simulink model "AMR_main_model_23b"  (R2023b)
settings: Solver=FixedStepAuto  StartTime=0.0  StopTime=inf  RelTol=1e-3
model workspace (MAT data in the model file):
  RTK_health_condition = 30
  mdlWSDbList = ["C:\Users\matlab.cut\Desktop\AMR\canbus_files\tramontina_database_mobotic.dbc" "C:\Users\matlab.cut\Desktop\AMR\canbus_files\tramontina_database_nvidia.dbc" "C:\Users\matlab.cut\Desktop\AMR\canbus_files\tramontina_database_sick_modbus.dbc" "C:\Users\matlab.cut\Desktop\AMR\canbus_files\tramontina_database_xsens.dbc" "tramontina_database_curtis.dbc"]
  min_motor_rpm = 30
  wheel_diameter = 360
undefined symbols (not defined in the file or in its folder): Down, Pull
libraries: speedgoatlib_IO60X_IO69X x12, tramontina_database_nvidialib x7, tramontina_database_curtislib x7, tramontina_database_xsenslib x4, speedgoatlib_IO691 x2, simulink x2, tramontina_database_sick_modbuslib x1, canmsglib x1
(part 1 of 2)
settings Model: Creator=matlab.cut  LastModifiedBy=matlab.cut
settings SolverCC: ConcurrentTasks=on  PositivePriorityOrder=on
settings OptimizationCC: BlockReduction=off  OptimizeBlockIOStorage=off
settings DebuggingCC: TasksWithSamePriorityMsg=none
settings HardwareCC: ProdBitPerLong=64  ProdLongLongMode=on  ProdHWDeviceType=Intel->x86-64 (Linux 64)
settings SFSimCC: MATLABDynamicMemAlloc=off
settings RTWCC: Description=Simulink Real-Time  SystemTargetFile=slrealtime.tlc  TemplateMakefile=slrealtime_default_tmf  Toolchain=Simulink Real-Time Toolchain  BuildConfiguration=Faster Runs  CodeExecutionProfiling=on  TargetLang=C++
settings CodeAppCC: MaxIdLength=127

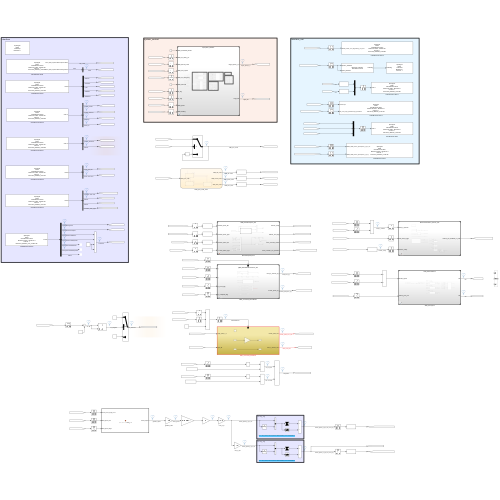
[thumbnail: Simulink's stored preview of the top-level diagram]
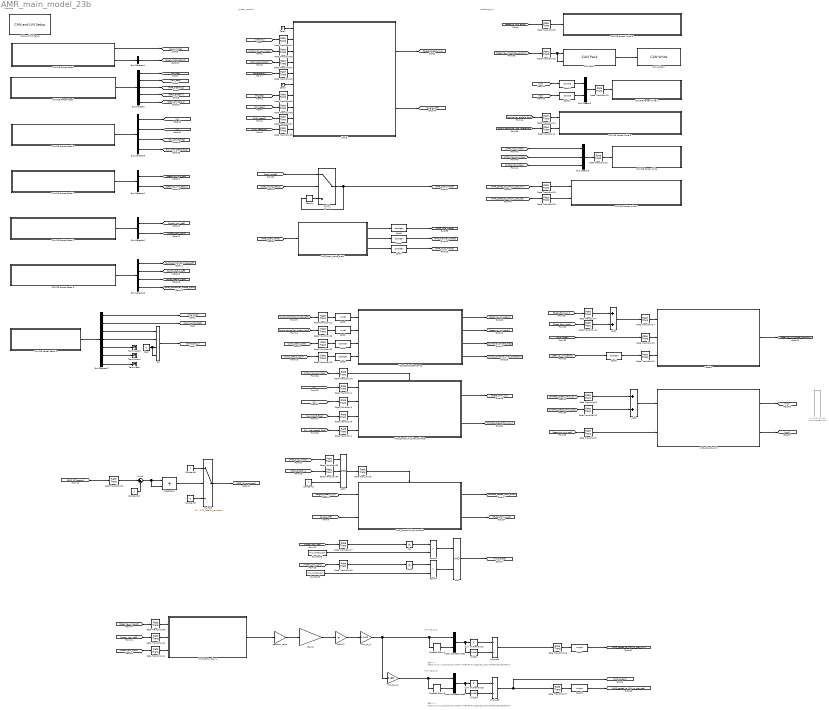
== system AMR_main_model_23b ==
  note: interface
  note: system_control
  note: interface_out
  note: REF ->> https://www.youtube.com/watch?v=BV3H-0wlcSs&ab_channel=EmbeddedRoom
  note: moving_avg
  note: REF ->> https://www.youtube.com/watch?v=BV3H-0wlcSs&ab_channel=EmbeddedRoom
  note: moving_avg
  AMR_ControlUnit_AutoMode : Subsystem  TreatAsAtomicUnit=on
  AMR_ControlUnit_ManualMode : ModelReference  ModelNameDialog=AMR_ManualModeControlUnit_23b.slx  SimulationMode=Normal  ModelReferenceVersion=1.33  EnablePortName=Enable  EnablePortStatesWhenEnabling=held
  AMR_VelocityUnit : ModelReference  ModelNameDialog=AMR_differentialDrive.slx  SimulationMode=Normal  ModelReferenceVersion=1.13
  AMR_oper_mode_chart : Stateflow chart  TreatAsAtomicUnit=on
  AND : Logic  AllPortsSameDT=off  OutDataTypeStr=boolean
  AND1 : Logic  Inputs=3  AllPortsSameDT=off  OutDataTypeStr=boolean
  Abs : Abs  SaturateOnIntegerOverflow=off
  Abs3 : Abs  SaturateOnIntegerOverflow=off
  Add1 : Sum
  Add2 : Sum
  Bus Creator2 : BusCreator  Inputs=2
  Bus Creator3 : BusCreator  Inputs=3
  Bus Selector : BusSelector  OutputSignals=ID113_LongLat.latitude,ID113_LongLat.longitude,ID34_EulerAngles.yaw,ID17_StatusWord.GNSSfix,ID17_StatusWord.RtkStatus
  Bus Selector1 : BusSelector  OutputSignals=ID288_mobotic_feedback_pos.position_feedback,ID288_mobotic_feedback_pos.MessageStatus.Status
  Bus Selector2 : BusSelector  OutputSignals=ID422_curtis_feedback_message_left.motor_rpm_left,ID423_curtis_feedback_message_right.motor_rpm_right
  Bus Selector4 : BusSelector  OutputSignals=Status  OutputAsBus=on
  Bus Selector5 : BusSelector  OutputSignals=ID368_joystick_axes.joystick_throttle,ID368_joystick_axes.joystick_direction,ID369_joystick_buttons.button_5,ID369_joystick_buttons.button_6
  Bus Selector6 : BusSelector  OutputSignals=ID1830_controller_status_left.controller_mode_left,ID1830_controller_status_left.MessageStatus.Status,ID1831_controller_status_right.MessageStatus.Status,ID1831_controller_status_right.controller_mode_right
  Bus Selector7 : BusSelector  OutputSignals=ID341_read_from_flexisoft.AuxEmEmergencia,ID341_read_from_flexisoft.AuxScannerInterrompido,ID341_read_from_flexisoft.EmergenciaFrontalDireita,ID341_read_from_flexisoft.EmergenciaFrontalEsquerda,ID341_read_from_flexisoft.EmergenciaTraseiraDireita,ID341_read_from_flexisoft.EmergenciaTraseiraEsquerda,ID341_read_from_flexisoft.MessageStatus.Status
  CAN DB Parser Read : Subsystem
      settings: OpenFcn=sg_can.OpenFcnRead;
      mask Help: eval('sg.utils.help.show(''io_main/refentry_ref_can_ofa_parsing_read'');')
      mask Display: disp('Speedgoat\nIO691\nCAN DB Parser Read\nModule ID: IO691 - Module ID 1\nChannel:  1\ntramontina_database_xsens.dbc ');
  "CAN DB Parser Read " : Subsystem
      settings: OpenFcn=sg_can.OpenFcnRead;
      mask Help: eval('sg.utils.help.show(''io_main/refentry_ref_can_ofa_parsing_read'');')
      mask Display: disp('Speedgoat\nIO691\nCAN DB Parser Read\nModule ID: IO691 - Module ID 1\nChannel:  1\ntramontina_database_nvidia.dbc ');
  CAN DB Parser Read 1 : Subsystem
      settings: OpenFcn=sg_can.OpenFcnRead;
      mask Help: eval('sg.utils.help.show(''io_main/refentry_ref_can_ofa_parsing_read'');')
      mask Display: disp('Speedgoat\nIO691\nCAN DB Parser Read\nModule ID: IO691 - Module ID 1\nChannel:  1\ntramontina_database_nvidia.dbc ');
  CAN DB Parser Read 2 : Subsystem
      settings: OpenFcn=sg_can.OpenFcnRead;
      mask Help: eval('sg.utils.help.show(''io_main/refentry_ref_can_ofa_parsing_read'');')
      mask Display: disp('Speedgoat\nIO691\nCAN DB Parser Read\nModule ID: IO691 - Module ID 1\nChannel:  1\ntramontina_database_curtis.dbc ');
  CAN DB Parser Read 3 : Subsystem
      settings: OpenFcn=sg_can.OpenFcnRead;
      mask Help: eval('sg.utils.help.show(''io_main/refentry_ref_can_ofa_parsing_read'');')
      mask Display: disp('Speedgoat\nIO691\nCAN DB Parser Read\nModule ID: IO691 - Module ID 1\nChannel:  1\ntramontina_database_curtis.dbc ');
  CAN DB Parser Read 5 : Subsystem
      settings: OpenFcn=sg_can.OpenFcnRead;
      mask Help: eval('sg.utils.help.show(''io_main/refentry_ref_can_ofa_parsing_read'');')
      mask Display: disp('Speedgoat\nIO691\nCAN DB Parser Read\nModule ID: IO691 - Module ID 1\nChannel:  1\ntramontina_database_nvidia.dbc ');
  CAN DB Parser Read 6 : Subsystem
      settings: OpenFcn=sg_can.OpenFcnRead;
      mask Help: eval('sg.utils.help.show(''io_main/refentry_ref_can_ofa_parsing_read'');')
      mask Display: disp('Speedgoat\nIO691\nCAN DB Parser Read\nModule ID: IO691 - Module ID 1\nChannel:  1\ntramontina_database_sick_modbus.dbc ');
  "CAN DB Parser Write " : Subsystem
      settings: OpenFcn=sg_can.OpenFcnWrite;
      mask Help: eval('sg.utils.help.show(''io_main/refentry_ref_can_ofa_parsing_write'');')
      mask Display: disp('Speedgoat\nIO691\nCAN DB Parser Write\nModule ID: IO691 - Module ID 1\nChannel:  1\ntramontina_database_nvidia.dbc ');
  CAN DB Parser Write 1 : Subsystem
      settings: OpenFcn=sg_can.OpenFcnWrite;
      mask Help: eval('sg.utils.help.show(''io_main/refentry_ref_can_ofa_parsing_write'');')
      mask Display: disp('Speedgoat\nIO691\nCAN DB Parser Write\nModule ID: IO691 - Module ID 1\nChannel:  1\ntramontina_database_nvidia.dbc ');
  CAN DB Parser Write 2 : Subsystem
      settings: OpenFcn=sg_can.OpenFcnWrite;
      mask Help: eval('sg.utils.help.show(''io_main/refentry_ref_can_ofa_parsing_write'');')
      mask Display: disp('Speedgoat\nIO691\nCAN DB Parser Write\nModule ID: IO691 - Module ID 1\nChannel:  1\ntramontina_database_curtis.dbc ');
  CAN DB Parser Write 3 : Subsystem
      settings: OpenFcn=sg_can.OpenFcnWrite;
      mask Help: eval('sg.utils.help.show(''io_main/refentry_ref_can_ofa_parsing_write'');')
      mask Display: disp('Speedgoat\nIO691\nCAN DB Parser Write\nModule ID: IO691 - Module ID 1\nChannel:  1\ntramontina_database_curtis.dbc ');
  CAN DB Parser Write 5 : Subsystem
      settings: OpenFcn=sg_can.OpenFcnWrite;
      mask Help: eval('sg.utils.help.show(''io_main/refentry_ref_can_ofa_parsing_write'');')
      mask Display: disp('Speedgoat\nIO691\nCAN DB Parser Write\nModule ID: IO691 - Module ID 1\nChannel:  1\ntramontina_database_nvidia.dbc ');
  CAN Pack2 : canmsglib/CAN Pack  MsgList=(none)  MsgName=CAN Msg  MsgIDType=Standard (11-bit identifier)  MsgIdentifier=0x120  MsgLength=8  Remote=off  ApplyMinMax=off  BusOutput=on  SignalInfo={ 'position_feedback', '0', '32', 'LE', 'signed', 'Standard', '0', '1', '0', '-inf', 'inf'; 'pulse_feedback', '32', '32', 'LE', 'signed', 'Standard', '0', '1', '0', '-Inf', 'Inf' }
      settings: DataFormat=manually specified signals
  CAN Write 2 : speedgoatlib_IO691/CAN Write   moduleType=IO691  id=1  channel=1  canType=CAN (HS)  messageType=CAN (HS)  useBusIn=on  numOfMsg=1  enableInput=off  enableStatusPort=off  ts=20e-3  initValues=[691 1 0.02 0 1 1 0 1 0 1]
      settings: SourceProductName=Simulink Real-Time: Speedgoat I/O Blockset
  "CAN and LIN Setup " : speedgoatlib_IO691/CAN and LIN Setup   moduleInitValues="[691    1    1   -1   -1]"  id=1  moduleType=IO691  pciSlot=-1  canChn1=CAN (HS)  canChn2=Disabled  canChn3=Disabled  canChn4=Disabled  linChn1=Disabled  linChn2=Disabled  canInitStructArray=[]  canTermStructArray=[]  gpioChnx=Disabled  canChn1InitValues="[2   2   8   1  16   3  19   2   2   5   2   0]"  arbBdrChn1=500 kBaud  clockDividerChn1=Enable  arbManBdrChn1=[8,1,16,3]  fdBdrChn1=5.0 MBaud  fdManBdrChn1=[2,2,5,2]  termResistor1=off  canChn2InitValues="[1   0   2   8  31   8  19   2   2   5   2   0]"  arbBdrChn2=1.0 MBaud  clockDividerChn2=Enable  arbManBdrChn2=[2,8,31,8]  fdBdrChn2=5.0 MBaud  fdManBdrChn2=[2,2,5,2]  termResistor2=off  canChn3InitValues="[1   0   2   8  31   8  19   2   2   5   2   0]"  arbBdrChn3=1.0 MBaud  clockDividerChn3=Enable  arbManBdrChn3=[2,8,31,8]  fdBdrChn3=5.0 MBaud  fdManBdrChn3=[2,2,5,2]  termResistor3=off  canChn4InitValues="[1   0   2   8  31   8  19   2   2   5   2   0]"  arbBdrChn4=1.0 MBaud  clockDividerChn4=Enable  arbManBdrChn4=[2,8,31,8]  fdBdrChn4=5.0 MBaud  fdManBdrChn4=[2,2,5,2]  termResistor4=off  linChn1InitValues="[0  9600]"  linBtrChn1=9600  linChn2InitValues="[0  9600]"  linBtrChn2=9600  doInitTermStruct="[0  5  0  0  0]"  parDoChannels=[1 2]  parDoVoltage=5  parDoInitValues=0  parDoReset=1  parNumOfDoS=0  parDiChannels=[3 4]  parDiVoltage=5  parDiPull=Pull-Down
      settings: LibrarySourceBlock=speedgoatlib_IO602_IO691/CAN and LIN Setup
  Cast1 : DataTypeConversion  OutDataTypeStr=single  SaturateOnIntegerOverflow=off  RndMeth=Floor
  Cast10 : DataTypeConversion  OutDataTypeStr=double  SaturateOnIntegerOverflow=off  RndMeth=Floor
  Cast11 : DataTypeConversion  OutDataTypeStr=double  SaturateOnIntegerOverflow=off  RndMeth=Floor
  Cast12 : DataTypeConversion  OutDataTypeStr=single  SaturateOnIntegerOverflow=off  RndMeth=Floor
  Cast2 : DataTypeConversion  OutDataTypeStr=uint8  SaturateOnIntegerOverflow=off  RndMeth=Floor
  Cast{3..4,6..9} (6 alike) : DataTypeConversion  OutDataTypeStr=boolean  SaturateOnIntegerOverflow=off  RndMeth=Floor
  Cast5 : DataTypeConversion  OutDataTypeStr=uint8  SaturateOnIntegerOverflow=off  RndMeth=Floor
  Constant1 : Constant
  Constant10 : Constant
  Constant3 : Constant  Value=min_motor_rpm
  Constant5 : Constant  Value=min_motor_rpm
  Constant8 : Constant
  Constant9 : Constant  Value=0
  Equal3 : RelationalOperator  Operator=>  OutDataTypeStr=boolean  RndMeth=Simplest  InputSameDT=off
  Equal4 : RelationalOperator  Operator=>  OutDataTypeStr=boolean  RndMeth=Simplest  InputSameDT=off
  Gain11 : Gain  Gain=pi
  Gain8 : Gain  Gain=wheel_diameter
  Integrator1 : Integrator  ExternalReset=either  UpperSaturationLimit=1  LowerSaturationLimit=0  WrappedStateUpperValue=30  WrappedStateLowerValue=0
  MATLAB Function1 : MATLAB Function  TreatAsAtomicUnit=on
  Memory : Memory  InheritSampleTime=on
  Model : ModelReference  ModelNameDialog=deployAGV_stateflow.slx  SimulationMode=Normal  ModelReferenceVersion=2.62
  Model2 : ModelReference  ModelNameDialog=MotorControllerDrive_mobotic_23b.slx  SimulationMode=Normal  ModelReferenceVersion=1.57
  MotorStartupSequence : ModelReference  ModelNameDialog=AMR_MotorStartupUnit_23b.slx  SimulationMode=Normal  ModelReferenceVersion=1.24
  Multiport Switch : MultiPortSwitch  Commented=on  DataPortOrder=Zero-based contiguous  Inputs=2  zeroidx=on  SaturateOnIntegerOverflow=off  InputSameDT=off
  OR : Logic  Operator=OR  Inputs=4  AllPortsSameDT=off  OutDataTypeStr=boolean
  Product1 : Product  Inputs=*/
  Product3 : Product  Inputs=*/
  Rate Transition{1..44} (44 alike) : RateTransition
  Sum of Elements1 : Sum  Inputs=+
  Sum of Elements3 : Sum  Inputs=+
  Sum1 : Sum  Inputs=|+-
  Switch : Switch  Criteria=u2 > Threshold  SaturateOnIntegerOverflow=off  InputSameDT=off
  Switch2 : Switch  Criteria=u2 > Threshold  Threshold=RTK_health_condition  SaturateOnIntegerOverflow=off  InputSameDT=off
  Tapped Delay1 : simulink/Discrete/Tapped Delay  vinit=0  samptime=-1  NumDelays=9  DelayOrder=Oldest  includeCurrent=off
  Tapped Delay3 : simulink/Discrete/Tapped Delay  vinit=0  samptime=-1  NumDelays=9  DelayOrder=Oldest  includeCurrent=off
  Terminator : Terminator
  Terminator1 : Terminator
  Terminator2 : Terminator
  Vector Concatenate1 : Concatenate
  Vector Concatenate3 : Concatenate
  Width1 : Width
  Width3 : Width
  Zero : Constant  Value=0  OutDataTypeStr=Inherit: Inherit via back propagation
  Zero1 : Constant  Value=0  OutDataTypeStr=Inherit: Inherit via back propagation
  Zero2 : Constant  Value=0  OutDataTypeStr=Inherit: Inherit via back propagation
  gearbox_ratio : Gain  Gain=1/40.61
  mm_to_m : Gain  Gain=1/1000
  mm_to_m1 : Gain  Gain=1/60
  wires:
  Zero2/1 -> Model/6
  [scanner_blocked] -> Rate Transition42/1
  [emergency] -> Rate Transition43/1
  Zero1/1 -> Model/1
  [interlock] -> Rate Transition44/1
  Bus Selector/3 -> [AMR_heading]  "<yaw>"
  [lat_deg] -> Rate Transition35/1
  OR/1 -> [emergency]  "emergency"
  [lon_deg] -> Rate Transition36/1
  [AMR_speed] -> Rate Transition37/1
  [AMR_heading] -> Rate Transition39/1
  [AMR_manual_mode] -> Rate Transition30/1
  Bus Selector7/1 -> [interlock]  "<AuxEmEmergencia>"
  Zero/1 -> OR/3, OR/4
  AMR_oper_mode_chart/2(AMR_manual_mode) -> Cast6/1  "AMR_manual_mode"
  Cast7/1 -> [AMR_auto_mode]
  Equal4/1 -> AND/2  "min_vel_right"
  AMR_ControlUnit_ManualMode/1 -> [theta_from_joy]  "theta_from_joy"
  [curtis_status_left] -> Rate Transition22/1
  Cast9/1 -> MotorStartupSequence/4
  Cast3/1 -> MotorStartupSequence/3
  [xj] -> Rate Transition1/1
  Cast5/1 -> MotorStartupSequence/1
  [throttle_speed_from_joy] -> Rate Transition8/1
  Add1/1 -> Rate Transition14/1  "theta_to_mobotic"
  AMR_ControlUnit_AutoMode/1(throttle_speed_auto) -> [throttle_speed_from_auto]  "throttle_speed_from_auto"
  Rate Transition18/1 -> Model2/2
  Rate Transition22/1 -> Cast3/1
  MotorStartupSequence/2 -> [steering_unit_error]
  Rate Transition21/1 -> Cast5/1
  Equal3/1 -> AND/1  "min_vel_left"
  [AMR_manual_mode] -> Rate Transition16/1
  [motor_rpm_right] -> Rate Transition13/1
  AMR_VelocityUnit/2 -> [rws]  "rws"
  Abs3/1 -> Equal4/1
  AMR_VelocityUnit/1 -> [lws]  "lws"
  Abs/1 -> Equal3/1
  Rate Transition16/1 -> AMR_ControlUnit_ManualMode/Enable
  AND/1 -> [hold_theta]  "hold_theta"
  Model2/1 -> [steering_unit_theta_position]
  [AMR_oper_mode] -> AMR_oper_mode_chart/1(AMR_oper_mode)
  [curtis_status_right] -> Rate Transition23/1
  [theta_from_joy] -> Rate Transition7/1
  [theta_from_auto] -> Rate Transition11/1
  Rate Transition7/1 -> Add1/1
  Rate Transition11/1 -> Add1/2
  Rate Transition4/1 -> AMR_ControlUnit_ManualMode/4
  Rate Transition8/1 -> Add2/1
  Rate Transition9/1 -> AMR_ControlUnit_AutoMode/Enable  "AutoModeActive"
  [curtis_controller_mode_right] -> Rate Transition20/1
  [steering_unit_ready] -> Cast4/1
  [curtis_controller_mode_left] -> Rate Transition21/1
  Rate Transition1/1 -> AMR_ControlUnit_ManualMode/1
  Rate Transition2/1 -> AMR_ControlUnit_ManualMode/2
  AND1/1 -> Rate Transition9/1
  AMR_ControlUnit_AutoMode/2(theta_to_mobotic_auto) -> [theta_from_auto]  "theta_from_auto"
  [oper_mode_status] -> Switch/2
  Rate Transition13/1 -> Abs3/1
  [oper_mode] -> Switch/1
  Cast4/1 -> Rate Transition19/1  "mobotic_ready"
  [joy_maxspeed_flag] -> Rate Transition4/1
  Rate Transition20/1 -> Cast2/1
  Rate Transition17/1 -> Abs/1
  Rate Transition3/1 -> AMR_ControlUnit_ManualMode/3
  Cast2/1 -> MotorStartupSequence/2
  MotorStartupSequence/4 -> [curtis_controller_into_operation]
  [yj] -> Rate Transition2/1
  [joy_boost_flag] -> Rate Transition3/1
  Rate Transition23/1 -> Cast9/1
  AMR_oper_mode_chart/1(AMR_idle_mode) -> Cast8/1  "AMR_idle_mode"
  Rate Transition19/1 -> Model2/3
  [motor_rpm_left] -> Rate Transition17/1
  MotorStartupSequence/3 -> [controller_enable_flag]
  Switch/1 -> [AMR_oper_mode], Memory/1  "AMR_oper_mode"
  Constant3/1 -> Equal4/2
  Rate Transition14/1 -> Model2/1
  Cast8/1 -> [AMR_idle_mode]
  Memory/1 -> Switch/3
  AMR_ControlUnit_ManualMode/2 -> [throttle_speed_from_joy]  "throttle_speed_from_joy"
  Constant5/1 -> Equal3/2
  [throttle_speed_from_auto] -> Rate Transition12/1
  [hold_theta] -> Rate Transition18/1
  AMR_oper_mode_chart/3(AMR_auto_mode) -> Cast7/1  "AMR_auto_mode"
  Add2/1 -> AMR_VelocityUnit/1
  [steering_unit_pos] -> Rate Transition5/1
  Rate Transition5/1 -> AMR_VelocityUnit/2
  MotorStartupSequence/1 -> [steering_unit_ready]
  Cast6/1 -> [AMR_manual_mode]
  [target_speed_m_s] -> AMR_ControlUnit_AutoMode/1(target_speed_m_s)
  "CAN DB Parser Read "/2(ID343_AMR_OperationMode.MessageStatus) -> Bus Selector4/1  "status"
  "CAN DB Parser Read "/1(ID343_AMR_OperationMode.OperationMode) -> [oper_mode]  "oper_mode"
  Bus Selector4/1 -> [oper_mode_status]  "status"
  Bus Selector5/1 -> [xj]  "<joystick_throttle>"
  Bus Selector5/4 -> [joy_maxspeed_flag]  "<button_6>"
  Bus Selector5/2 -> [yj]  "<joystick_direction>"
  Bus Selector5/3 -> [joy_boost_flag]  "<button_5>"
  CAN DB Parser Read 5/1(CAN Rx) -> Bus Selector5/1
  Bus Selector1/1 -> [steering_unit_pos]  "<position_feedback>"
  CAN DB Parser Read 1/1(CAN Rx) -> Bus Selector1/1
  Bus Selector1/2 -> [steering_unit_status]  "<Status>"
  Bus Selector6/3 -> [curtis_status_right]  "<Status>"
  Bus Selector6/4 -> [curtis_controller_mode_right]  "<controller_mode_right>"
  Bus Selector2/2 -> [motor_rpm_right]  "<motor_rpm_right>"
  Bus Selector6/1 -> [curtis_controller_mode_left]  "<controller_mode_left>"
  Bus Selector2/1 -> [motor_rpm_left]  "<motor_rpm_left>"
  Bus Selector6/2 -> [curtis_status_left]  "<Status>"
  CAN DB Parser Read 3/1(CAN Rx) -> Bus Selector6/1
  CAN DB Parser Read 2/1(CAN Rx) -> Bus Selector2/1
  Rate Transition25/1 -> "CAN DB Parser Write "/1(CAN Tx)
  [rws] -> Cast11/1  "rws"
  [AMR_auto_mode] -> Bus Creator3/3
  Rate Transition24/1 -> CAN DB Parser Write 3/1(Enable Input)
  Bus Creator3/1 -> Rate Transition25/1
  [AMR_manual_mode] -> Bus Creator3/2
  Bus Creator2/1 -> Rate Transition15/1
  Rate Transition10/1 -> CAN Pack2/2, CAN Pack2/1
  [AMR_idle_mode] -> Bus Creator3/1
  Cast11/1 -> Bus Creator2/2
  Cast10/1 -> Bus Creator2/1
  Rate Transition15/1 -> CAN DB Parser Write 2/1(CAN Tx)
  [curtis_controller_into_operation] -> Rate Transition6/1
  [lws] -> Cast10/1  "lws"
  [steering_unit_theta_position] -> Rate Transition10/1
  [controller_enable_flag] -> Rate Transition24/1
  CAN Pack2/1 -> CAN Write 2/1
  Rate Transition6/1 -> CAN DB Parser Write 3/2(ID0_curtis_input_operational.pre_operational)
  [steering_unit_error] -> Rate Transition32/1
  Model/2 -> [angle_diff]  "angle_diff"
  [angle_diff] -> AMR_ControlUnit_AutoMode/2(angle_diff)
  Bus Selector7/4 -> OR/2  "<EmergenciaFrontalEsquerda>"
  Bus Selector7/2 -> [scanner_blocked]  "<AuxScannerInterrompido>"
  Bus Selector7/7 -> Terminator/1  "<Status>"
  Bus Selector7/3 -> OR/1  "<EmergenciaFrontalDireita>"
  CAN DB Parser Read 6/1(CAN Rx) -> Bus Selector7/1
  Bus Selector7/6 -> Terminator1/1  "<EmergenciaTraseiraEsquerda>"
  Bus Selector7/5 -> Terminator2/1  "<EmergenciaTraseiraDireita>"
  Model/1 -> [target_speed_m_s]  "target_speed_m_s"
  CAN DB Parser Read/1(CAN Rx) -> Bus Selector/1
  Bus Selector/1 -> [lat_deg]  "<latitude>"
  Bus Selector/2 -> [lon_deg]  "<longitude>"
  Bus Selector/4 -> [GPS_GNSSfix]  "<GNSSfix>"
  Bus Selector/5 -> [GPS_RTKstatus]  "<RtkStatus>"
  [GPS_RTKstatus] -> Rate Transition31/1
  [GPS_GNSSfix] -> Rate Transition34/1
  [AMR_auto_mode] -> Rate Transition33/1
  Constant1/1 -> AND1/3
  Constant8/1 -> Switch2/1
  Switch2/1 -> [GPS_rtk_trustness]  "rtk_trustness"
  Integrator1/1 -> Switch2/2  "rtk_integrator"
  Sum1/1 -> Integrator1/2, Integrator1/1  "rtk_diff"
  Constant9/1 -> Switch2/3
  Constant10/1 -> Sum1/2
  [steering_unit_pos] -> Rate Transition38/1
  [motor_rpm_left] -> Rate Transition40/1
  [motor_rpm_right] -> Rate Transition41/1
  gearbox_ratio/1 -> Gain8/1  "wheel_speed"
  Rate Transition40/1 -> MATLAB Function1/2(RPM_Speed_Left)
  Rate Transition38/1 -> MATLAB Function1/1(Actual_Curve_Angle_Front)
  Gain8/1 -> Gain11/1
  Rate Transition41/1 -> MATLAB Function1/3(RPM_Speed_Right)
  MATLAB Function1/1(Vehicle_Speed) -> gearbox_ratio/1  "gearbox_speed"
  Gain11/1 -> mm_to_m/1
  Cast12/1 -> [AMR_speed_to_CAN_m_per_sec]
  Rate Transition26/1 -> Cast1/1
  Cast1/1 -> [AMR_speed_to_CAN_m_per_min]
  Rate Transition27/1 -> Cast12/1
  Sum of Elements3/1 -> Product3/1
  mm_to_m1/1 -> Tapped Delay3/1, Vector Concatenate3/1  "vehicle_speed_m_per_sec"
  Product3/1 -> [AMR_speed], Rate Transition27/1  "vehicle_speed_m_per_sec_mov_avg"
  Width3/1 -> Product3/2
  Vector Concatenate3/1 -> Width3/1, Sum of Elements3/1
  Tapped Delay3/1 -> Vector Concatenate3/2
  Tapped Delay1/1 -> Vector Concatenate1/2
  Width1/1 -> Product1/2
  Sum of Elements1/1 -> Product1/1
  Product1/1 -> Rate Transition26/1  "vehicle_speed_m_per_min_mov_avg"
  Vector Concatenate1/1 -> Sum of Elements1/1, Width1/1
  mm_to_m/1 -> mm_to_m1/1, Tapped Delay1/1, Vector Concatenate1/1  "vehicle_speed_m_per_min"
  [AMR_speed_to_CAN_m_per_min] -> Rate Transition28/1
  [AMR_speed_to_CAN_m_per_sec] -> Rate Transition29/1
  Rate Transition28/1 -> CAN DB Parser Write 1/1(ID290_AMR_vehicle_speed.speed_m_per_min)
  Rate Transition29/1 -> CAN DB Parser Write 1/2(ID290_AMR_vehicle_speed.speed_m_per_s)
  Rate Transition30/1 -> Model/3
  Rate Transition31/1 -> Sum1/1
  Rate Transition32/1 -> CAN DB Parser Write 5/1(ID289_mobotic_error_flag.steering_unit_error)
  Rate Transition33/1 -> AND1/1
  Rate Transition34/1 -> AND1/2
  Rate Transition35/1 -> Model/7
  Rate Transition36/1 -> Model/8
  Rate Transition37/1 -> Model/9
  Rate Transition39/1 -> Model/10
  Rate Transition42/1 -> Model/4
  Rate Transition43/1 -> Model/5
  Rate Transition44/1 -> Model/2
  Rate Transition12/1 -> Add2/2

== system AMR_main_model_23b/AMR_ControlUnit_AutoMode ==
  target_speed_m_s : Inport
  angle_diff : Inport  Port=2
  Enable : EnablePort  OutDataTypeStr=boolean
  gearbox_ratio : Gain  Gain=40.61
  throttle_speed_auto : Outport  OutputWhenDisabled=reset  InitialOutput=[0]
  theta_to_mobotic_auto : Outport  Port=2  OutputWhenDisabled=reset  InitialOutput=[0]
  wires:
  target_speed_m_s/1 -> gearbox_ratio/1
  angle_diff/1 -> theta_to_mobotic_auto/1
  gearbox_ratio/1 -> throttle_speed_auto/1

== system AMR_main_model_23b/CAN DB Parser Read ==
  ReadSubsystem : Subsystem
  UnpackSubsystem : Subsystem
  CAN Rx : Outport
  wires:
  ReadSubsystem/1(Raw_Rx) -> UnpackSubsystem/1(Unpack_In)
  ReadSubsystem/2(Status_Rx) -> UnpackSubsystem/2(Status Inport)
  UnpackSubsystem/1(Unpack_Out) -> CAN Rx/1

== system AMR_main_model_23b/CAN DB Parser Read  ==
  ReadSubsystem : Subsystem
  SelectSignal_1_1 : BusSelector  OutputSignals=ID343_AMR_OperationMode.OperationMode
  SelectStatus_1 : BusSelector  OutputSignals=ID343_AMR_OperationMode.MessageStatus
  UnpackSubsystem : Subsystem
  ID343_AMR_OperationMode.OperationMode : Outport
  ID343_AMR_OperationMode.MessageStatus : Outport  Port=2
  wires:
  ReadSubsystem/1(Raw_Rx) -> UnpackSubsystem/1(Unpack_In)
  ReadSubsystem/2(Status_Rx) -> UnpackSubsystem/2(Status Inport)
  UnpackSubsystem/1(Unpack_Out) -> SelectSignal_1_1/1, SelectStatus_1/1
  SelectSignal_1_1/1 -> ID343_AMR_OperationMode.OperationMode/1  "<OperationMode>"
  SelectStatus_1/1 -> ID343_AMR_OperationMode.MessageStatus/1  "<MessageStatus>"

== system AMR_main_model_23b/CAN DB Parser Read 1 ==
  ReadSubsystem : Subsystem
  UnpackSubsystem : Subsystem
  CAN Rx : Outport
  wires:
  ReadSubsystem/1(Raw_Rx) -> UnpackSubsystem/1(Unpack_In)
  ReadSubsystem/2(Status_Rx) -> UnpackSubsystem/2(Status Inport)
  UnpackSubsystem/1(Unpack_Out) -> CAN Rx/1

== system AMR_main_model_23b/CAN DB Parser Read 2 ==
  ReadSubsystem : Subsystem
  UnpackSubsystem : Subsystem
  CAN Rx : Outport
  wires:
  ReadSubsystem/1(Raw_Rx) -> UnpackSubsystem/1(Unpack_In)
  ReadSubsystem/2(Status_Rx) -> UnpackSubsystem/2(Status Inport)
  UnpackSubsystem/1(Unpack_Out) -> CAN Rx/1

== system AMR_main_model_23b/CAN DB Parser Read 3 ==
  ReadSubsystem : Subsystem
  UnpackSubsystem : Subsystem
  CAN Rx : Outport
  wires:
  ReadSubsystem/1(Raw_Rx) -> UnpackSubsystem/1(Unpack_In)
  ReadSubsystem/2(Status_Rx) -> UnpackSubsystem/2(Status Inport)
  UnpackSubsystem/1(Unpack_Out) -> CAN Rx/1

== system AMR_main_model_23b/CAN DB Parser Read 5 ==
  ReadSubsystem : Subsystem
  UnpackSubsystem : Subsystem
  CAN Rx : Outport
  wires:
  ReadSubsystem/1(Raw_Rx) -> UnpackSubsystem/1(Unpack_In)
  ReadSubsystem/2(Status_Rx) -> UnpackSubsystem/2(Status Inport)
  UnpackSubsystem/1(Unpack_Out) -> CAN Rx/1

== system AMR_main_model_23b/CAN DB Parser Read 6 ==
  ReadSubsystem : Subsystem
  UnpackSubsystem : Subsystem
  CAN Rx : Outport
  wires:
  ReadSubsystem/1(Raw_Rx) -> UnpackSubsystem/1(Unpack_In)
  ReadSubsystem/2(Status_Rx) -> UnpackSubsystem/2(Status Inport)
  UnpackSubsystem/1(Unpack_Out) -> CAN Rx/1

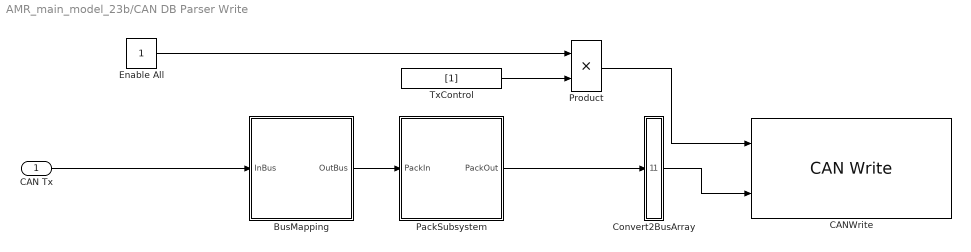
== system AMR_main_model_23b/CAN DB Parser Write  ==
  CAN Tx : Inport
  BusMapping : Subsystem
  CANWrite : speedgoatlib_IO60X_IO69X/CAN/CAN Write   moduleType=IO691  id=1  channel=1  canType=CAN (HS)  messageType=CAN (HS)  useBusIn=on  numOfMsg=1  enableInput=on  enableStatusPort=off  ts=500e-3  initValues=[691 1 0.5 0 1 1 0 1 1 1]
  Convert2BusArray : Subsystem
  Enable All : Constant  OutDataTypeStr=boolean
  PackSubsystem : Subsystem
  Product : Product  OutDataTypeStr=uint32
  TxControl : Constant  Value=[1]  OutDataTypeStr=uint32
  wires:
  PackSubsystem/1(PackOut) -> Convert2BusArray/1(InBus)
  Convert2BusArray/1(BusArrayOut) -> CANWrite/2
  Product/1 -> CANWrite/1
  TxControl/1 -> Product/2
  Enable All/1 -> Product/1
  CAN Tx/1 -> BusMapping/1(InBus)
  BusMapping/1(OutBus) -> PackSubsystem/1(PackIn)

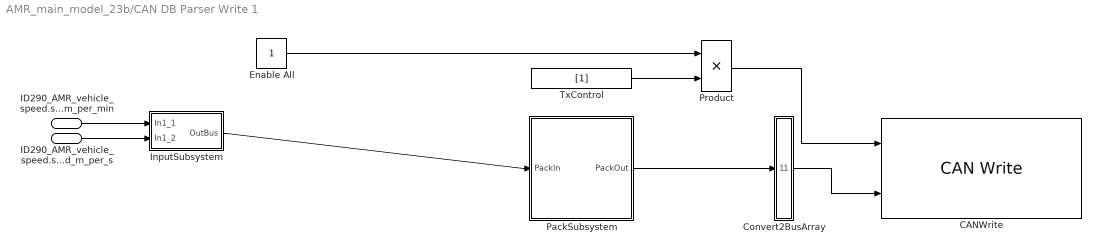
== system AMR_main_model_23b/CAN DB Parser Write 1 ==
  ID290_AMR_vehicle_speed.speed_m_per_min : Inport
  ID290_AMR_vehicle_speed.speed_m_per_s : Inport  Port=2
  CANWrite : speedgoatlib_IO60X_IO69X/CAN/CAN Write   moduleType=IO691  id=1  channel=1  canType=CAN (HS)  messageType=CAN (HS)  useBusIn=on  numOfMsg=1  enableInput=on  enableStatusPort=off  ts=50e-3  initValues=[691 1 0.05 0 1 1 0 1 1 1]
  Convert2BusArray : Subsystem
  Enable All : Constant  OutDataTypeStr=boolean
  InputSubsystem : Subsystem
  PackSubsystem : Subsystem
  Product : Product  OutDataTypeStr=uint32
  TxControl : Constant  Value=[1]  OutDataTypeStr=uint32
  wires:
  PackSubsystem/1(PackOut) -> Convert2BusArray/1(InBus)
  Convert2BusArray/1(BusArrayOut) -> CANWrite/2
  Product/1 -> CANWrite/1
  TxControl/1 -> Product/2
  Enable All/1 -> Product/1
  ID290_AMR_vehicle_speed.speed_m_per_min/1 -> InputSubsystem/1(In1_1)
  ID290_AMR_vehicle_speed.speed_m_per_s/1 -> InputSubsystem/2(In1_2)
  InputSubsystem/1(OutBus) -> PackSubsystem/1(PackIn)

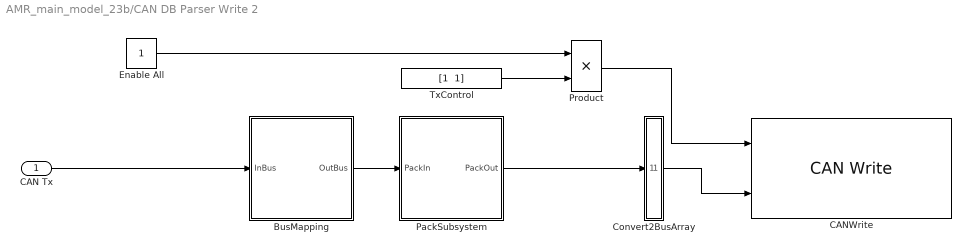
== system AMR_main_model_23b/CAN DB Parser Write 2 ==
  CAN Tx : Inport
  BusMapping : Subsystem
  CANWrite : speedgoatlib_IO60X_IO69X/CAN/CAN Write   moduleType=IO691  id=1  channel=1  canType=CAN (HS)  messageType=CAN (HS)  useBusIn=on  numOfMsg=2  enableInput=on  enableStatusPort=off  ts=10e-3  initValues=[691 1 0.01 0 1 1 0 2 1 1]
  Convert2BusArray : Subsystem
  Enable All : Constant  OutDataTypeStr=boolean
  PackSubsystem : Subsystem
  Product : Product  OutDataTypeStr=uint32
  TxControl : Constant  Value="[1  1]"  OutDataTypeStr=uint32
  wires:
  PackSubsystem/1(PackOut) -> Convert2BusArray/1(InBus)
  Convert2BusArray/1(BusArrayOut) -> CANWrite/2
  Product/1 -> CANWrite/1
  TxControl/1 -> Product/2
  Enable All/1 -> Product/1
  CAN Tx/1 -> BusMapping/1(InBus)
  BusMapping/1(OutBus) -> PackSubsystem/1(PackIn)

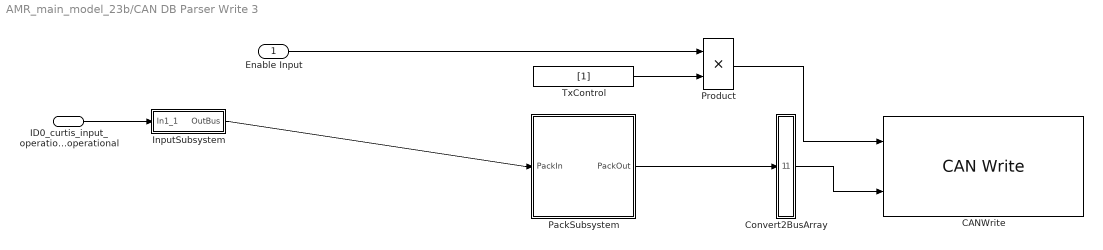
== system AMR_main_model_23b/CAN DB Parser Write 3 ==
  Enable Input : Inport  OutDataTypeStr=boolean
  ID0_curtis_input_operational.pre_operational : Inport  Port=2
  CANWrite : speedgoatlib_IO60X_IO69X/CAN/CAN Write   moduleType=IO691  id=1  channel=1  canType=CAN (HS)  messageType=CAN (HS)  useBusIn=on  numOfMsg=1  enableInput=on  enableStatusPort=off  ts=500e-3  initValues=[691 1 0.5 0 1 1 0 1 1 1]
  Convert2BusArray : Subsystem
  InputSubsystem : Subsystem
  PackSubsystem : Subsystem
  Product : Product  OutDataTypeStr=uint32
  TxControl : Constant  Value=[1]  OutDataTypeStr=uint32
  wires:
  PackSubsystem/1(PackOut) -> Convert2BusArray/1(InBus)
  Convert2BusArray/1(BusArrayOut) -> CANWrite/2
  Product/1 -> CANWrite/1
  TxControl/1 -> Product/2
  Enable Input/1 -> Product/1
  ID0_curtis_input_operational.pre_operational/1 -> InputSubsystem/1(In1_1)
  InputSubsystem/1(OutBus) -> PackSubsystem/1(PackIn)

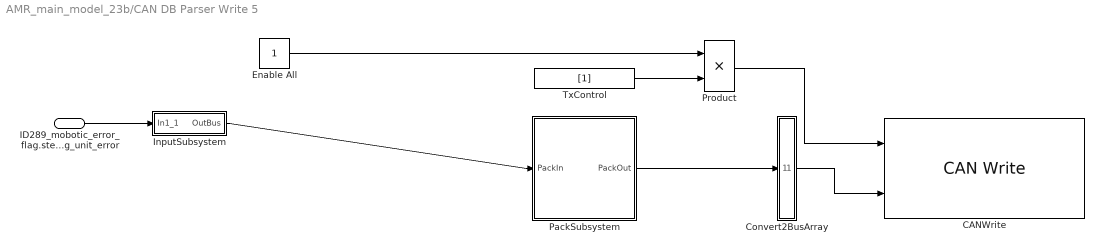
== system AMR_main_model_23b/CAN DB Parser Write 5 ==
  ID289_mobotic_error_flag.steering_unit_error : Inport
  CANWrite : speedgoatlib_IO60X_IO69X/CAN/CAN Write   moduleType=IO691  id=1  channel=1  canType=CAN (HS)  messageType=CAN (HS)  useBusIn=on  numOfMsg=1  enableInput=on  enableStatusPort=off  ts=500e-3  initValues=[691 1 0.5 0 1 1 0 1 1 1]
  Convert2BusArray : Subsystem
  Enable All : Constant  OutDataTypeStr=boolean
  InputSubsystem : Subsystem
  PackSubsystem : Subsystem
  Product : Product  OutDataTypeStr=uint32
  TxControl : Constant  Value=[1]  OutDataTypeStr=uint32
  wires:
  PackSubsystem/1(PackOut) -> Convert2BusArray/1(InBus)
  Convert2BusArray/1(BusArrayOut) -> CANWrite/2
  Product/1 -> CANWrite/1
  TxControl/1 -> Product/2
  Enable All/1 -> Product/1
  ID289_mobotic_error_flag.steering_unit_error/1 -> InputSubsystem/1(In1_1)
  InputSubsystem/1(OutBus) -> PackSubsystem/1(PackIn)

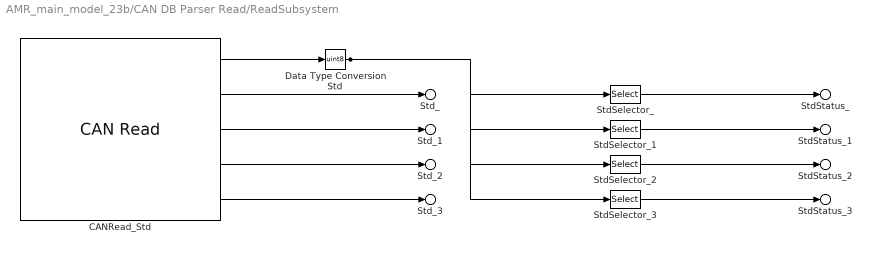
== system AMR_main_model_23b/CAN DB Parser Read/ReadSubsystem ==
  CANRead_Std : speedgoatlib_IO60X_IO69X/CAN/CAN Read   moduleType=IO691  id=1  channel=1  canType=CAN (HS)  messageType=CAN (HS)  useBusOut=on  HasMulRead=Specify by IDs  MsgIDlist="[17   34  113  118]"  isEFF=off  LabelInHex=off  enableInput=off  initValues=[691 1 0.005 0 1 1 0 1 2 0 4 17 34 113 118]  ts=5e-3
  Data Type ConversionStd : DataTypeConversion  OutDataTypeStr=uint8  SaturateOnIntegerOverflow=off  RndMeth=Floor
  StdSelector_ : Selector  IndexOptions=Index vector (dialog)  Indices=1  OutputSizes=1
  StdSelector_1 : Selector  IndexOptions=Index vector (dialog)  Indices=2  OutputSizes=1
  StdSelector_2 : Selector  IndexOptions=Index vector (dialog)  Indices=3  OutputSizes=1
  StdSelector_3 : Selector  IndexOptions=Index vector (dialog)  Indices=4  OutputSizes=1
  Std_ : Outport  PortName=Raw_Rx  Element=Std.ID17
  Std_1 : Outport  PortName=Raw_Rx  Element=Std.ID34
  Std_2 : Outport  PortName=Raw_Rx  Element=Std.ID113
  Std_3 : Outport  PortName=Raw_Rx  Element=Std.ID118
  StdStatus_ : Outport  Port=2  PortName=Status_Rx  Element=Std.ID17
  StdStatus_1 : Outport  Port=2  PortName=Status_Rx  Element=Std.ID34
  StdStatus_2 : Outport  Port=2  PortName=Status_Rx  Element=Std.ID113
  StdStatus_3 : Outport  Port=2  PortName=Status_Rx  Element=Std.ID118
  wires:
  CANRead_Std/1 -> Data Type ConversionStd/1
  CANRead_Std/2 -> Std_/1
  CANRead_Std/3 -> Std_1/1
  CANRead_Std/4 -> Std_2/1
  CANRead_Std/5 -> Std_3/1
  Data Type ConversionStd/1 -> StdSelector_/1, StdSelector_1/1, StdSelector_2/1, StdSelector_3/1
  StdSelector_/1 -> StdStatus_/1
  StdSelector_1/1 -> StdStatus_1/1
  StdSelector_2/1 -> StdStatus_2/1
  StdSelector_3/1 -> StdStatus_3/1

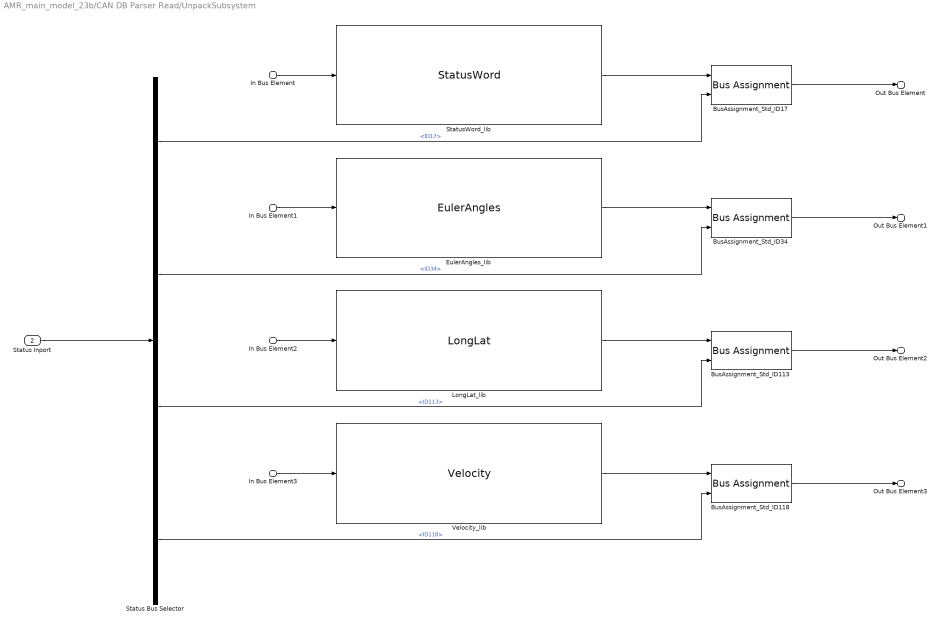
== system AMR_main_model_23b/CAN DB Parser Read/UnpackSubsystem ==
  In Bus Element : Inport  PortName=Unpack_In  Element=Std.ID17
  In Bus Element1 : Inport  PortName=Unpack_In  Element=Std.ID34
  In Bus Element2 : Inport  PortName=Unpack_In  Element=Std.ID113
  In Bus Element3 : Inport  PortName=Unpack_In  Element=Std.ID118
  Status Inport : Inport  Port=2
  BusAssignment_Std_ID{17,34,113,118} (4 alike) : BusAssignment  AssignedSignals=MessageStatus.Status
  EulerAngles_lib : tramontina_database_xsenslib/CAN unpack/EulerAngles  SystemSampleTime=-1  VariantActivationTime=update diagram  AllowFlexibleInterface=on  Latency=0  AutoFrameSizeCalculation=off
  LongLat_lib : tramontina_database_xsenslib/CAN unpack/LongLat  SystemSampleTime=-1  VariantActivationTime=update diagram  AllowFlexibleInterface=on  Latency=0  AutoFrameSizeCalculation=off
  Status Bus Selector : BusSelector  OutputSignals=Std.ID17,Std.ID34,Std.ID113,Std.ID118
  StatusWord_lib : tramontina_database_xsenslib/CAN unpack/StatusWord  SystemSampleTime=-1  VariantActivationTime=update diagram  AllowFlexibleInterface=on  Latency=0  AutoFrameSizeCalculation=off
  Velocity_lib : tramontina_database_xsenslib/CAN unpack/Velocity  SystemSampleTime=-1  VariantActivationTime=update diagram  AllowFlexibleInterface=on  Latency=0  AutoFrameSizeCalculation=off
  Out Bus Element : Outport  PortName=Unpack_Out  Element=ID17_StatusWord
  Out Bus Element1 : Outport  PortName=Unpack_Out  Element=ID34_EulerAngles
  Out Bus Element2 : Outport  PortName=Unpack_Out  Element=ID113_LongLat
  Out Bus Element3 : Outport  PortName=Unpack_Out  Element=ID118_Velocity
  wires:
  In Bus Element/1 -> StatusWord_lib/1
  StatusWord_lib/1 -> BusAssignment_Std_ID17/1
  BusAssignment_Std_ID17/1 -> Out Bus Element/1
  In Bus Element1/1 -> EulerAngles_lib/1
  EulerAngles_lib/1 -> BusAssignment_Std_ID34/1
  BusAssignment_Std_ID34/1 -> Out Bus Element1/1
  In Bus Element2/1 -> LongLat_lib/1
  LongLat_lib/1 -> BusAssignment_Std_ID113/1
  BusAssignment_Std_ID113/1 -> Out Bus Element2/1
  In Bus Element3/1 -> Velocity_lib/1
  Velocity_lib/1 -> BusAssignment_Std_ID118/1
  BusAssignment_Std_ID118/1 -> Out Bus Element3/1
  Status Inport/1 -> Status Bus Selector/1
  Status Bus Selector/1 -> BusAssignment_Std_ID17/2  "<ID17>"
  Status Bus Selector/2 -> BusAssignment_Std_ID34/2  "<ID34>"
  Status Bus Selector/3 -> BusAssignment_Std_ID113/2  "<ID113>"
  Status Bus Selector/4 -> BusAssignment_Std_ID118/2  "<ID118>"

== system AMR_main_model_23b/CAN DB Parser Read /ReadSubsystem ==
  CANRead_Std : speedgoatlib_IO60X_IO69X/CAN/CAN Read   moduleType=IO691  id=1  channel=1  canType=CAN (HS)  messageType=CAN (HS)  useBusOut=on  HasMulRead=Specify by IDs  MsgIDlist=[343]  isEFF=off  LabelInHex=off  enableInput=off  initValues=[691 1 0.05 0 1 1 0 1 2 0 1 343]  ts=50e-3
  Data Type ConversionStd : DataTypeConversion  OutDataTypeStr=uint8  SaturateOnIntegerOverflow=off  RndMeth=Floor
  StdSelector_ : Selector  IndexOptions=Index vector (dialog)  Indices=1  OutputSizes=1
  Std_ : Outport  PortName=Raw_Rx  Element=Std.ID343
  StdStatus_ : Outport  Port=2  PortName=Status_Rx  Element=Std.ID343
  wires:
  CANRead_Std/1 -> Data Type ConversionStd/1
  CANRead_Std/2 -> Std_/1
  Data Type ConversionStd/1 -> StdSelector_/1
  StdSelector_/1 -> StdStatus_/1

== system AMR_main_model_23b/CAN DB Parser Read /UnpackSubsystem ==
  In Bus Element : Inport  PortName=Unpack_In  Element=Std.ID343
  Status Inport : Inport  Port=2
  AMR_OperationMode_lib : tramontina_database_nvidialib/CAN unpack/AMR_OperationMode  SystemSampleTime=-1  VariantActivationTime=update diagram  AllowFlexibleInterface=on  Latency=0  AutoFrameSizeCalculation=off
  BusAssignment_Std_ID343 : BusAssignment  AssignedSignals=MessageStatus.Status
  Status Bus Selector : BusSelector  OutputSignals=Std.ID343
  Out Bus Element : Outport  PortName=Unpack_Out  Element=ID343_AMR_OperationMode
  wires:
  In Bus Element/1 -> AMR_OperationMode_lib/1
  AMR_OperationMode_lib/1 -> BusAssignment_Std_ID343/1
  BusAssignment_Std_ID343/1 -> Out Bus Element/1
  Status Inport/1 -> Status Bus Selector/1
  Status Bus Selector/1 -> BusAssignment_Std_ID343/2  "<ID343>"

== system AMR_main_model_23b/CAN DB Parser Read 1/ReadSubsystem ==
  CANRead_Std : speedgoatlib_IO60X_IO69X/CAN/CAN Read   moduleType=IO691  id=1  channel=1  canType=CAN (HS)  messageType=CAN (HS)  useBusOut=on  HasMulRead=Specify by IDs  MsgIDlist=[288]  isEFF=off  LabelInHex=off  enableInput=off  initValues=[691 1 0.005 0 1 1 0 1 2 0 1 288]  ts=5e-3
  Data Type ConversionStd : DataTypeConversion  OutDataTypeStr=uint8  SaturateOnIntegerOverflow=off  RndMeth=Floor
  StdSelector_ : Selector  IndexOptions=Index vector (dialog)  Indices=1  OutputSizes=1
  Std_ : Outport  PortName=Raw_Rx  Element=Std.ID288
  StdStatus_ : Outport  Port=2  PortName=Status_Rx  Element=Std.ID288
  wires:
  CANRead_Std/1 -> Data Type ConversionStd/1
  CANRead_Std/2 -> Std_/1
  Data Type ConversionStd/1 -> StdSelector_/1
  StdSelector_/1 -> StdStatus_/1

== system AMR_main_model_23b/CAN DB Parser Read 1/UnpackSubsystem ==
  In Bus Element : Inport  PortName=Unpack_In  Element=Std.ID288
  Status Inport : Inport  Port=2
  BusAssignment_Std_ID288 : BusAssignment  AssignedSignals=MessageStatus.Status
  Status Bus Selector : BusSelector  OutputSignals=Std.ID288
  mobotic_feedback_pos_lib : tramontina_database_nvidialib/CAN unpack/mobotic_feedback_pos  SystemSampleTime=-1  VariantActivationTime=update diagram  AllowFlexibleInterface=on  Latency=0  AutoFrameSizeCalculation=off
  Out Bus Element : Outport  PortName=Unpack_Out  Element=ID288_mobotic_feedback_pos
  wires:
  In Bus Element/1 -> mobotic_feedback_pos_lib/1
  mobotic_feedback_pos_lib/1 -> BusAssignment_Std_ID288/1
  BusAssignment_Std_ID288/1 -> Out Bus Element/1
  Status Inport/1 -> Status Bus Selector/1
  Status Bus Selector/1 -> BusAssignment_Std_ID288/2  "<ID288>"

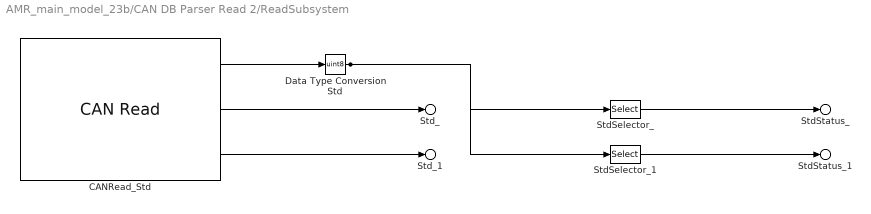
== system AMR_main_model_23b/CAN DB Parser Read 2/ReadSubsystem ==
  CANRead_Std : speedgoatlib_IO60X_IO69X/CAN/CAN Read   moduleType=IO691  id=1  channel=1  canType=CAN (HS)  messageType=CAN (HS)  useBusOut=on  HasMulRead=Specify by IDs  MsgIDlist="[422  423]"  isEFF=off  LabelInHex=off  enableInput=off  initValues=[691 1 0.05 0 1 1 0 1 2 0 2 422 423]  ts=50e-3
  Data Type ConversionStd : DataTypeConversion  OutDataTypeStr=uint8  SaturateOnIntegerOverflow=off  RndMeth=Floor
  StdSelector_ : Selector  IndexOptions=Index vector (dialog)  Indices=1  OutputSizes=1
  StdSelector_1 : Selector  IndexOptions=Index vector (dialog)  Indices=2  OutputSizes=1
  Std_ : Outport  PortName=Raw_Rx  Element=Std.ID422
  Std_1 : Outport  PortName=Raw_Rx  Element=Std.ID423
  StdStatus_ : Outport  Port=2  PortName=Status_Rx  Element=Std.ID422
  StdStatus_1 : Outport  Port=2  PortName=Status_Rx  Element=Std.ID423
  wires:
  CANRead_Std/1 -> Data Type ConversionStd/1
  CANRead_Std/2 -> Std_/1
  CANRead_Std/3 -> Std_1/1
  Data Type ConversionStd/1 -> StdSelector_/1, StdSelector_1/1
  StdSelector_/1 -> StdStatus_/1
  StdSelector_1/1 -> StdStatus_1/1

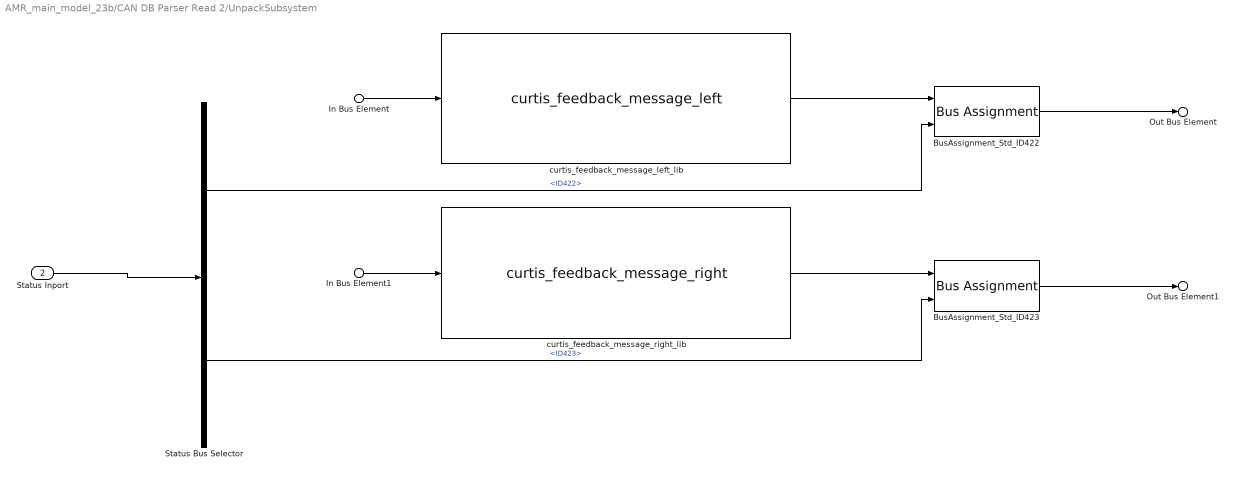
== system AMR_main_model_23b/CAN DB Parser Read 2/UnpackSubsystem ==
  In Bus Element : Inport  PortName=Unpack_In  Element=Std.ID422
  In Bus Element1 : Inport  PortName=Unpack_In  Element=Std.ID423
  Status Inport : Inport  Port=2
  BusAssignment_Std_ID422 : BusAssignment  AssignedSignals=MessageStatus.Status
  BusAssignment_Std_ID423 : BusAssignment  AssignedSignals=MessageStatus.Status
  Status Bus Selector : BusSelector  OutputSignals=Std.ID422,Std.ID423
  curtis_feedback_message_left_lib : tramontina_database_curtislib/CAN unpack/curtis_feedback_message_left  SystemSampleTime=-1  VariantActivationTime=update diagram  AllowFlexibleInterface=on  Latency=0  AutoFrameSizeCalculation=off
  curtis_feedback_message_right_lib : tramontina_database_curtislib/CAN unpack/curtis_feedback_message_right  SystemSampleTime=-1  VariantActivationTime=update diagram  AllowFlexibleInterface=on  Latency=0  AutoFrameSizeCalculation=off
  Out Bus Element : Outport  PortName=Unpack_Out  Element=ID422_curtis_feedback_message_left
  Out Bus Element1 : Outport  PortName=Unpack_Out  Element=ID423_curtis_feedback_message_right
  wires:
  In Bus Element/1 -> curtis_feedback_message_left_lib/1
  curtis_feedback_message_left_lib/1 -> BusAssignment_Std_ID422/1
  BusAssignment_Std_ID422/1 -> Out Bus Element/1
  In Bus Element1/1 -> curtis_feedback_message_right_lib/1
  curtis_feedback_message_right_lib/1 -> BusAssignment_Std_ID423/1
  BusAssignment_Std_ID423/1 -> Out Bus Element1/1
  Status Inport/1 -> Status Bus Selector/1
  Status Bus Selector/1 -> BusAssignment_Std_ID422/2  "<ID422>"
  Status Bus Selector/2 -> BusAssignment_Std_ID423/2  "<ID423>"

== system AMR_main_model_23b/CAN DB Parser Read 3/ReadSubsystem ==
  CANRead_Std : speedgoatlib_IO60X_IO69X/CAN/CAN Read   moduleType=IO691  id=1  channel=1  canType=CAN (HS)  messageType=CAN (HS)  useBusOut=on  HasMulRead=Specify by IDs  MsgIDlist="[1830  1831]"  isEFF=off  LabelInHex=off  enableInput=off  initValues=[691 1 0.5 0 1 1 0 1 2 0 2 1830 1831]  ts=500e-3
  Data Type ConversionStd : DataTypeConversion  OutDataTypeStr=uint8  SaturateOnIntegerOverflow=off  RndMeth=Floor
  StdSelector_ : Selector  IndexOptions=Index vector (dialog)  Indices=1  OutputSizes=1
  StdSelector_1 : Selector  IndexOptions=Index vector (dialog)  Indices=2  OutputSizes=1
  Std_ : Outport  PortName=Raw_Rx  Element=Std.ID1830
  Std_1 : Outport  PortName=Raw_Rx  Element=Std.ID1831
  StdStatus_ : Outport  Port=2  PortName=Status_Rx  Element=Std.ID1830
  StdStatus_1 : Outport  Port=2  PortName=Status_Rx  Element=Std.ID1831
  wires:
  CANRead_Std/1 -> Data Type ConversionStd/1
  CANRead_Std/2 -> Std_/1
  CANRead_Std/3 -> Std_1/1
  Data Type ConversionStd/1 -> StdSelector_/1, StdSelector_1/1
  StdSelector_/1 -> StdStatus_/1
  StdSelector_1/1 -> StdStatus_1/1

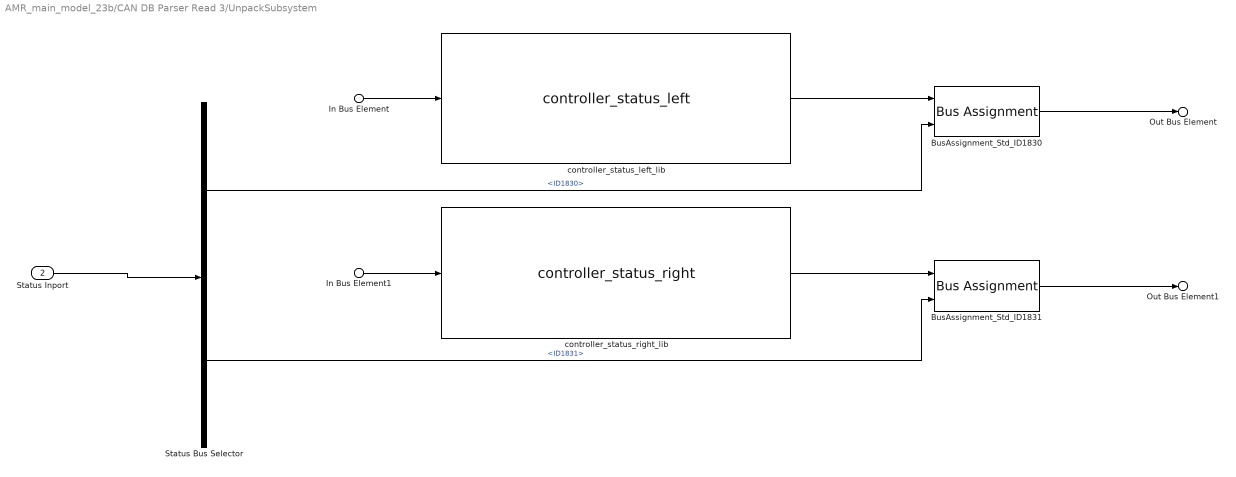
== system AMR_main_model_23b/CAN DB Parser Read 3/UnpackSubsystem ==
  In Bus Element : Inport  PortName=Unpack_In  Element=Std.ID1830
  In Bus Element1 : Inport  PortName=Unpack_In  Element=Std.ID1831
  Status Inport : Inport  Port=2
  BusAssignment_Std_ID1830 : BusAssignment  AssignedSignals=MessageStatus.Status
  BusAssignment_Std_ID1831 : BusAssignment  AssignedSignals=MessageStatus.Status
  Status Bus Selector : BusSelector  OutputSignals=Std.ID1830,Std.ID1831
  controller_status_left_lib : tramontina_database_curtislib/CAN unpack/controller_status_left  SystemSampleTime=-1  VariantActivationTime=update diagram  AllowFlexibleInterface=on  Latency=0  AutoFrameSizeCalculation=off
  controller_status_right_lib : tramontina_database_curtislib/CAN unpack/controller_status_right  SystemSampleTime=-1  VariantActivationTime=update diagram  AllowFlexibleInterface=on  Latency=0  AutoFrameSizeCalculation=off
  Out Bus Element : Outport  PortName=Unpack_Out  Element=ID1830_controller_status_left
  Out Bus Element1 : Outport  PortName=Unpack_Out  Element=ID1831_controller_status_right
  wires:
  In Bus Element/1 -> controller_status_left_lib/1
  controller_status_left_lib/1 -> BusAssignment_Std_ID1830/1
  BusAssignment_Std_ID1830/1 -> Out Bus Element/1
  In Bus Element1/1 -> controller_status_right_lib/1
  controller_status_right_lib/1 -> BusAssignment_Std_ID1831/1
  BusAssignment_Std_ID1831/1 -> Out Bus Element1/1
  Status Inport/1 -> Status Bus Selector/1
  Status Bus Selector/1 -> BusAssignment_Std_ID1830/2  "<ID1830>"
  Status Bus Selector/2 -> BusAssignment_Std_ID1831/2  "<ID1831>"

== system AMR_main_model_23b/CAN DB Parser Read 5/ReadSubsystem ==
  CANRead_Std : speedgoatlib_IO60X_IO69X/CAN/CAN Read   moduleType=IO691  id=1  channel=1  canType=CAN (HS)  messageType=CAN (HS)  useBusOut=on  HasMulRead=Specify by IDs  MsgIDlist="[368  369]"  isEFF=off  LabelInHex=off  enableInput=off  initValues=[691 1 0.01 0 1 1 0 1 2 0 2 368 369]  ts=10e-3
  Data Type ConversionStd : DataTypeConversion  OutDataTypeStr=uint8  SaturateOnIntegerOverflow=off  RndMeth=Floor
  StdSelector_ : Selector  IndexOptions=Index vector (dialog)  Indices=1  OutputSizes=1
  StdSelector_1 : Selector  IndexOptions=Index vector (dialog)  Indices=2  OutputSizes=1
  Std_ : Outport  PortName=Raw_Rx  Element=Std.ID368
  Std_1 : Outport  PortName=Raw_Rx  Element=Std.ID369
  StdStatus_ : Outport  Port=2  PortName=Status_Rx  Element=Std.ID368
  StdStatus_1 : Outport  Port=2  PortName=Status_Rx  Element=Std.ID369
  wires:
  CANRead_Std/1 -> Data Type ConversionStd/1
  CANRead_Std/2 -> Std_/1
  CANRead_Std/3 -> Std_1/1
  Data Type ConversionStd/1 -> StdSelector_/1, StdSelector_1/1
  StdSelector_/1 -> StdStatus_/1
  StdSelector_1/1 -> StdStatus_1/1

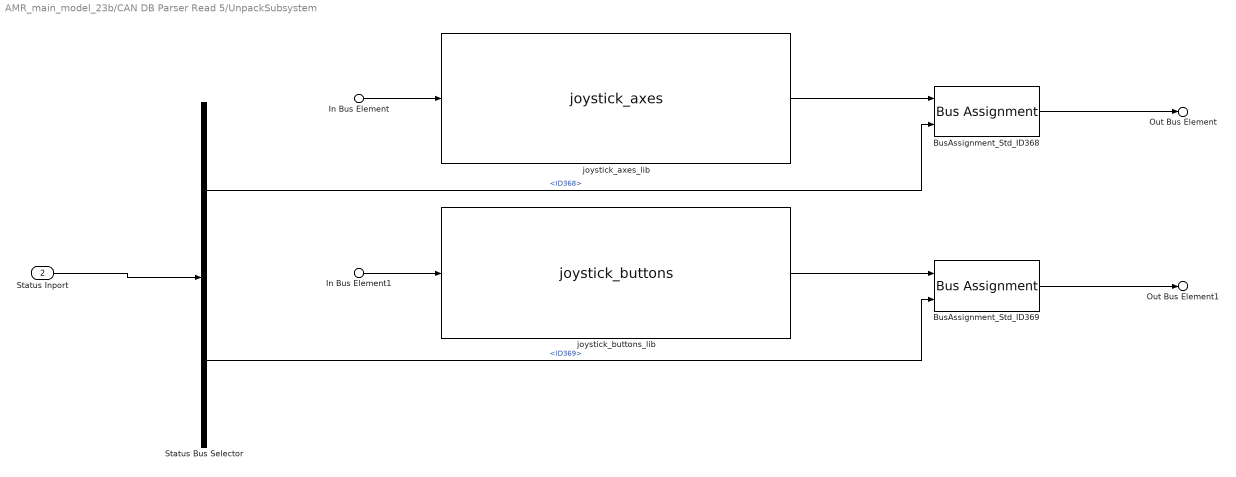
== system AMR_main_model_23b/CAN DB Parser Read 5/UnpackSubsystem ==
  In Bus Element : Inport  PortName=Unpack_In  Element=Std.ID368
  In Bus Element1 : Inport  PortName=Unpack_In  Element=Std.ID369
  Status Inport : Inport  Port=2
  BusAssignment_Std_ID368 : BusAssignment  AssignedSignals=MessageStatus.Status
  BusAssignment_Std_ID369 : BusAssignment  AssignedSignals=MessageStatus.Status
  Status Bus Selector : BusSelector  OutputSignals=Std.ID368,Std.ID369
  joystick_axes_lib : tramontina_database_nvidialib/CAN unpack/joystick_axes  SystemSampleTime=-1  VariantActivationTime=update diagram  AllowFlexibleInterface=on  Latency=0  AutoFrameSizeCalculation=off
  joystick_buttons_lib : tramontina_database_nvidialib/CAN unpack/joystick_buttons  SystemSampleTime=-1  VariantActivationTime=update diagram  AllowFlexibleInterface=on  Latency=0  AutoFrameSizeCalculation=off
  Out Bus Element : Outport  PortName=Unpack_Out  Element=ID368_joystick_axes
  Out Bus Element1 : Outport  PortName=Unpack_Out  Element=ID369_joystick_buttons
  wires:
  In Bus Element/1 -> joystick_axes_lib/1
  joystick_axes_lib/1 -> BusAssignment_Std_ID368/1
  BusAssignment_Std_ID368/1 -> Out Bus Element/1
  In Bus Element1/1 -> joystick_buttons_lib/1
  joystick_buttons_lib/1 -> BusAssignment_Std_ID369/1
  BusAssignment_Std_ID369/1 -> Out Bus Element1/1
  Status Inport/1 -> Status Bus Selector/1
  Status Bus Selector/1 -> BusAssignment_Std_ID368/2  "<ID368>"
  Status Bus Selector/2 -> BusAssignment_Std_ID369/2  "<ID369>"

== system AMR_main_model_23b/CAN DB Parser Read 6/ReadSubsystem ==
  CANRead_Std : speedgoatlib_IO60X_IO69X/CAN/CAN Read   moduleType=IO691  id=1  channel=1  canType=CAN (HS)  messageType=CAN (HS)  useBusOut=on  HasMulRead=Specify by IDs  MsgIDlist=[341]  isEFF=off  LabelInHex=off  enableInput=off  initValues=[691 1 0.1 0 1 1 0 1 2 0 1 341]  ts=100e-3
  Data Type ConversionStd : DataTypeConversion  OutDataTypeStr=uint8  SaturateOnIntegerOverflow=off  RndMeth=Floor
  StdSelector_ : Selector  IndexOptions=Index vector (dialog)  Indices=1  OutputSizes=1
  Std_ : Outport  PortName=Raw_Rx  Element=Std.ID341
  StdStatus_ : Outport  Port=2  PortName=Status_Rx  Element=Std.ID341
  wires:
  CANRead_Std/1 -> Data Type ConversionStd/1
  CANRead_Std/2 -> Std_/1
  Data Type ConversionStd/1 -> StdSelector_/1
  StdSelector_/1 -> StdStatus_/1

== system AMR_main_model_23b/CAN DB Parser Read 6/UnpackSubsystem ==
  In Bus Element : Inport  PortName=Unpack_In  Element=Std.ID341
  Status Inport : Inport  Port=2
  BusAssignment_Std_ID341 : BusAssignment  AssignedSignals=MessageStatus.Status
  Status Bus Selector : BusSelector  OutputSignals=Std.ID341
  read_from_flexisoft_lib : tramontina_database_sick_modbuslib/CAN unpack/read_from_flexisoft  SystemSampleTime=-1  VariantActivationTime=update diagram  AllowFlexibleInterface=on  Latency=0  AutoFrameSizeCalculation=off
  Out Bus Element : Outport  PortName=Unpack_Out  Element=ID341_read_from_flexisoft
  wires:
  In Bus Element/1 -> read_from_flexisoft_lib/1
  read_from_flexisoft_lib/1 -> BusAssignment_Std_ID341/1
  BusAssignment_Std_ID341/1 -> Out Bus Element/1
  Status Inport/1 -> Status Bus Selector/1
  Status Bus Selector/1 -> BusAssignment_Std_ID341/2  "<ID341>"

== system AMR_main_model_23b/CAN DB Parser Write /BusMapping ==
  signal3 : Inport  PortName=InBus  Element=signal3
  signal1 : Inport  PortName=InBus  Element=signal1
  signal2 : Inport  PortName=InBus  Element=signal2
  ID344_AMR_OperationMode_feedback.OperationMode_auto : Outport  PortName=OutBus  Element=ID344_AMR_OperationMode_feedback.OperationMode_auto
  ID344_AMR_OperationMode_feedback.OperationMode_idle : Outport  PortName=OutBus  Element=ID344_AMR_OperationMode_feedback.OperationMode_idle
  ID344_AMR_OperationMode_feedback.OperationMode_manual : Outport  PortName=OutBus  Element=ID344_AMR_OperationMode_feedback.OperationMode_manual
  wires:
  signal3/1 -> ID344_AMR_OperationMode_feedback.OperationMode_auto/1
  signal1/1 -> ID344_AMR_OperationMode_feedback.OperationMode_idle/1
  signal2/1 -> ID344_AMR_OperationMode_feedback.OperationMode_manual/1

== system AMR_main_model_23b/CAN DB Parser Write /Convert2BusArray ==
  In1 : Inport  PortName=InBus  Element=ID344_AMR_OperationMode_feedback
  BusArray : Concatenate  NumInputs=1
  BusArrayOut : Outport
  wires:
  In1/1 -> BusArray/1
  BusArray/1 -> BusArrayOut/1

== system AMR_main_model_23b/CAN DB Parser Write /PackSubsystem ==
  In Bus Element : Inport  PortName=PackIn  Element=ID344_AMR_OperationMode_feedback
  AMR_OperationMode_feedback_lib : tramontina_database_nvidialib/CAN pack/AMR_OperationMode_feedback  SystemSampleTime=-1  VariantActivationTime=update diagram  AllowFlexibleInterface=on  Latency=0  AutoFrameSizeCalculation=off
  In Bus Element1 : Outport  PortName=PackOut  Element=ID344_AMR_OperationMode_feedback
  wires:
  In Bus Element/1 -> AMR_OperationMode_feedback_lib/1
  AMR_OperationMode_feedback_lib/1 -> In Bus Element1/1

== system AMR_main_model_23b/CAN DB Parser Write 1/Convert2BusArray ==
  In1 : Inport  PortName=InBus  Element=ID290_AMR_vehicle_speed
  BusArray : Concatenate  NumInputs=1
  BusArrayOut : Outport
  wires:
  In1/1 -> BusArray/1
  BusArray/1 -> BusArrayOut/1

== system AMR_main_model_23b/CAN DB Parser Write 1/InputSubsystem ==
  In1_1 : Inport
  In1_2 : Inport  Port=2
  ID290_AMR_vehicle_speed.speed_m_per_min : Outport  PortName=OutBus  Element=ID290_AMR_vehicle_speed.speed_m_per_min
  ID290_AMR_vehicle_speed.speed_m_per_s : Outport  PortName=OutBus  Element=ID290_AMR_vehicle_speed.speed_m_per_s
  wires:
  In1_1/1 -> ID290_AMR_vehicle_speed.speed_m_per_min/1
  In1_2/1 -> ID290_AMR_vehicle_speed.speed_m_per_s/1
